simulink model "P5_Simulink"  (R2023a)
settings: Solver=ode23  StartTime=0.0  StopTime=0.005  RelTol=1e-3
values from neighbouring files (symbols this model uses):
  C = 0.1e-6    (= 1e-07)    [P5_RLC.m]    (also in P5_RLC_fig.m)
  L = 6e-3    (= 0.006)    [P5_RLC.m]
  R = 100    [P5_RLC.m]
settings Model: Creator=karen  LastModifiedBy=karen

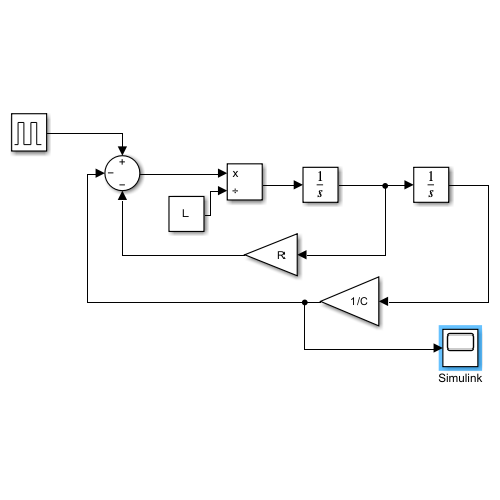
[thumbnail: Simulink's stored preview of the top-level diagram]
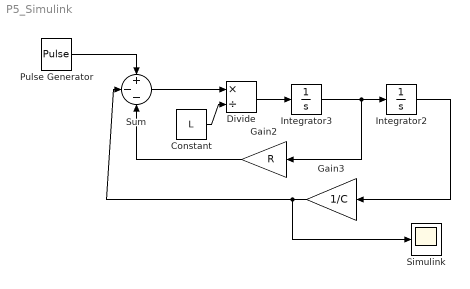
== system P5_Simulink ==
  Constant : Constant  Value=L
  Divide : Product  Inputs=*/
  Gain2 : Gain  Gain=R
  Gain3 : Gain  Gain=1/C
  Integrator2 : Integrator
  Integrator3 : Integrator
  Pulse Generator : DiscretePulseGenerator  PulseType=Time based  Amplitude=12  Period=2e-3  PulseWidth=50
  Simulink : Scope
  Sum : Sum  Inputs=+--
  wires:
  Integrator2/1 -> Gain3/1
  Integrator3/1 -> Gain2/1, Integrator2/1
  Constant/1 -> Divide/2
  Divide/1 -> Integrator3/1
  Sum/1 -> Divide/1
  Gain2/1 -> Sum/3
  Gain3/1 -> Simulink/1, Sum/2
  Pulse Generator/1 -> Sum/1
